simulink model "ps2actualmodel"  (R2022a)
settings: Solver=VariableStepAuto  StartTime=0.0  StopTime=10.0  RelTol=1e-3
settings Model: PacingRate=0.350000  Creator=StealthyPanda  LastModifiedBy=StealthyPanda

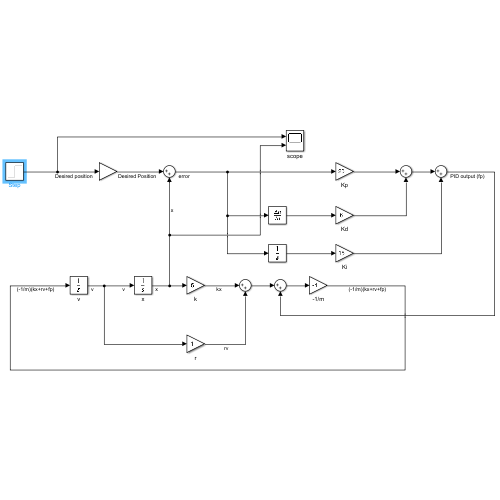
[thumbnail: Simulink's stored preview of the top-level diagram]
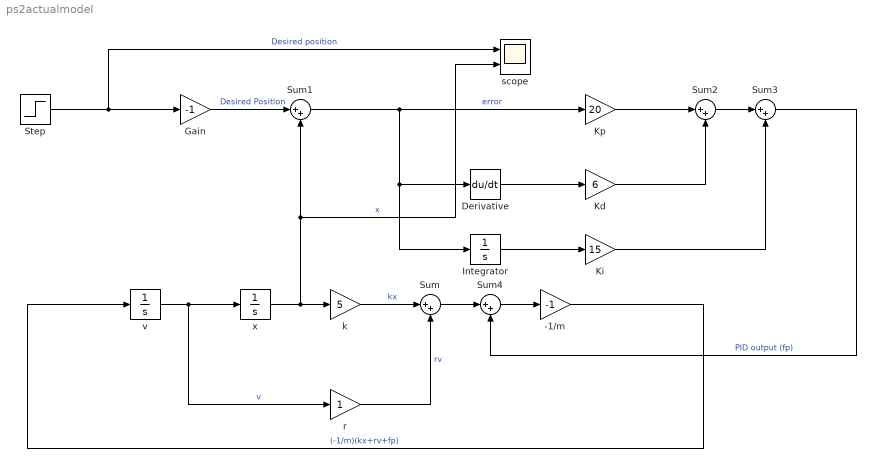
== system ps2actualmodel ==
  -1/m : Gain  Gain=-1
  Derivative : Derivative
  Gain : Gain  Gain=-1
  Integrator : Integrator
  Kd : Gain  Gain=6
  Ki : Gain  Gain=15
  Kp : Gain  Gain=20
  Step : Step  SampleTime=0
  Sum{,1..4} (5 alike) : Sum  Inputs=|++
  k : Gain  Gain=5
  r : Gain
  scope : Scope  NumInputPorts=2
  v : Integrator
  x : Integrator
  wires:
  x/1 -> scope/2, Sum1/2, k/1  "x"
  v/1 -> r/1, x/1  "v"
  r/1 -> Sum/2  "rv"
  k/1 -> Sum/1  "kx"
  -1/m/1 -> v/1  "(-1/m)(kx+rv+fp)"
  Step/1 -> scope/1, Gain/1  "Desired position"
  Sum1/1 -> Integrator/1, Derivative/1, Kp/1  "error"
  Integrator/1 -> Ki/1
  Derivative/1 -> Kd/1
  Kp/1 -> Sum2/1
  Kd/1 -> Sum2/2
  Sum2/1 -> Sum3/1
  Ki/1 -> Sum3/2
  Sum/1 -> Sum4/1
  Sum4/1 -> -1/m/1
  Gain/1 -> Sum1/1  "Desired Position"
  Sum3/1 -> Sum4/2  "PID output (fp)"
